simulink model "clark_bianhuan"  (R2024b)
settings: Solver=VariableStepAuto  StartTime=0.0  StopTime=0.4  RelTol=1e-3
settings Model: Creator=罗芳成  LastModifiedBy=罗芳成

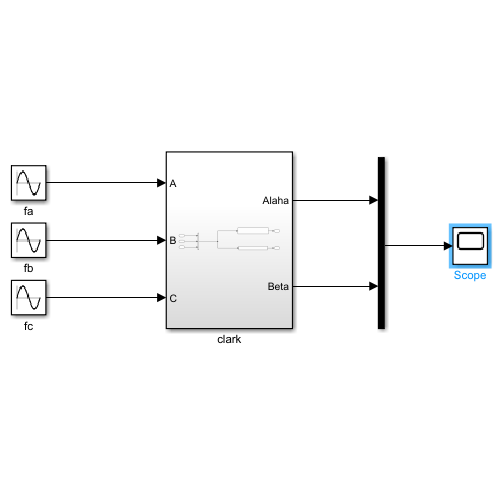
[thumbnail: Simulink's stored preview of the top-level diagram]
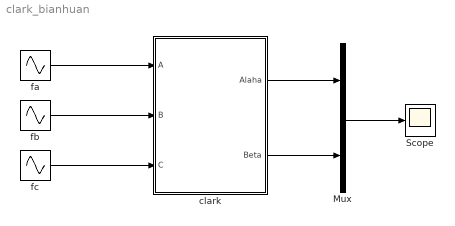
== system clark_bianhuan ==
  Mux : Mux  Inputs=2
  Scope : Scope
  clark : Subsystem
  fa : Sin  Amplitude=100  Frequency=100*pi  SampleTime=0
  fb : Sin  Amplitude=100  Frequency=100*pi  Phase=-2*pi/3  SampleTime=0
  fc : Sin  Amplitude=100  Frequency=100*pi  Phase=2*pi/3  SampleTime=0
  wires:
  fa/1 -> clark/1(A)
  fb/1 -> clark/2(B)
  fc/1 -> clark/3(C)
  clark/1(Alaha) -> Mux/1
  clark/2(Beta) -> Mux/2
  Mux/1 -> Scope/1

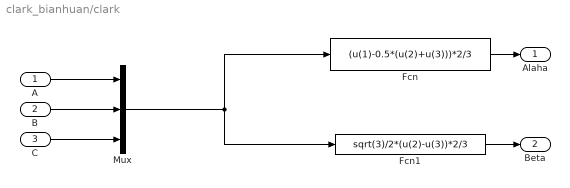
== system clark_bianhuan/clark ==
  A : Inport
  B : Inport  Port=2
  C : Inport  Port=3
  Fcn : Fcn  Expr=(u(1)-0.5*(u(2)+u(3)))*2/3
  Fcn1 : Fcn  Expr=sqrt(3)/2*(u(2)-u(3))*2/3
  Mux : Mux  Inputs=3
  Alaha : Outport
  Beta : Outport  Port=2
  wires:
  Fcn/1 -> Alaha/1
  C/1 -> Mux/3
  Fcn1/1 -> Beta/1
  B/1 -> Mux/2
  Mux/1 -> Fcn1/1, Fcn/1
  A/1 -> Mux/1
